simulink model "Rocket"  (R2020a)
settings: Solver=ode4  StartTime=0.0  StopTime=50000  FixedStep=0.5  RelTol=1e-3
undefined symbols (not defined in the file or in its folder): HDBK, MIL
libraries: powerlib_meascontrol x8, simulink x4, aerolibatmos2 x2
settings Model: Creator=j90xb  LastModifiedBy=jasch

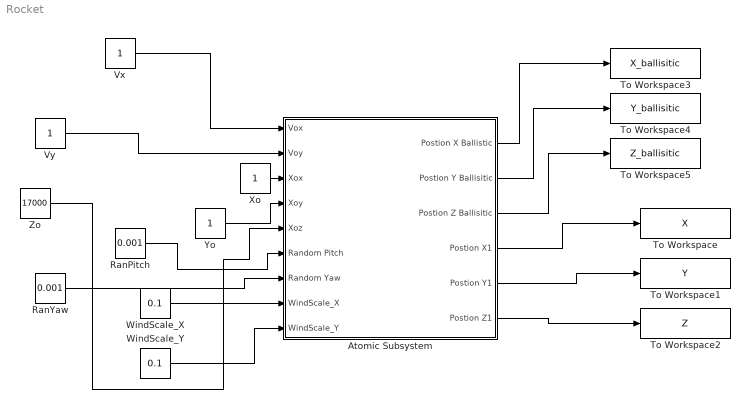
== system Rocket ==
  Atomic Subsystem : Subsystem  TreatAsAtomicUnit=on
  RanPitch : Constant  Value=0.001
  RanYaw : Constant  Value=0.001
  To Workspace : ToWorkspace  VariableName=X  SampleTime=-1
  To Workspace1 : ToWorkspace  VariableName=Y  SampleTime=-1
  To Workspace2 : ToWorkspace  VariableName=Z  SampleTime=-1
  To Workspace3 : ToWorkspace  VariableName=X_ballisitic  SampleTime=-1
  To Workspace4 : ToWorkspace  VariableName=Y_ballisitic  SampleTime=-1
  To Workspace5 : ToWorkspace  VariableName=Z_ballisitic  SampleTime=-1
  Vx : Constant
  Vy : Constant
  WindScale_X : Constant  Value=0.1
  WindScale_Y : Constant  Value=0.1
  Xo : Constant
  Yo : Constant
  Zo : Constant  Value=17000
  wires:
  Vx/1 -> Atomic Subsystem/1(Vox)
  Zo/1 -> Atomic Subsystem/5(Xoz)
  Atomic Subsystem/4(Postion X1) -> To Workspace/1
  Atomic Subsystem/5(Postion Y1) -> To Workspace1/1
  Atomic Subsystem/6(Postion Z1) -> To Workspace2/1
  Atomic Subsystem/1(Postion X Ballistic) -> To Workspace3/1
  Atomic Subsystem/2(Postion Y Ballisitic) -> To Workspace4/1
  Atomic Subsystem/3(Postion Z Ballisitic) -> To Workspace5/1
  Vy/1 -> Atomic Subsystem/2(Voy)
  Xo/1 -> Atomic Subsystem/3(Xox)
  Yo/1 -> Atomic Subsystem/4(Xoy)
  RanPitch/1 -> Atomic Subsystem/6(Random Pitch)
  RanYaw/1 -> Atomic Subsystem/7(Random Yaw)
  WindScale_X/1 -> Atomic Subsystem/8(WindScale_X)
  WindScale_Y/1 -> Atomic Subsystem/9(WindScale_Y)

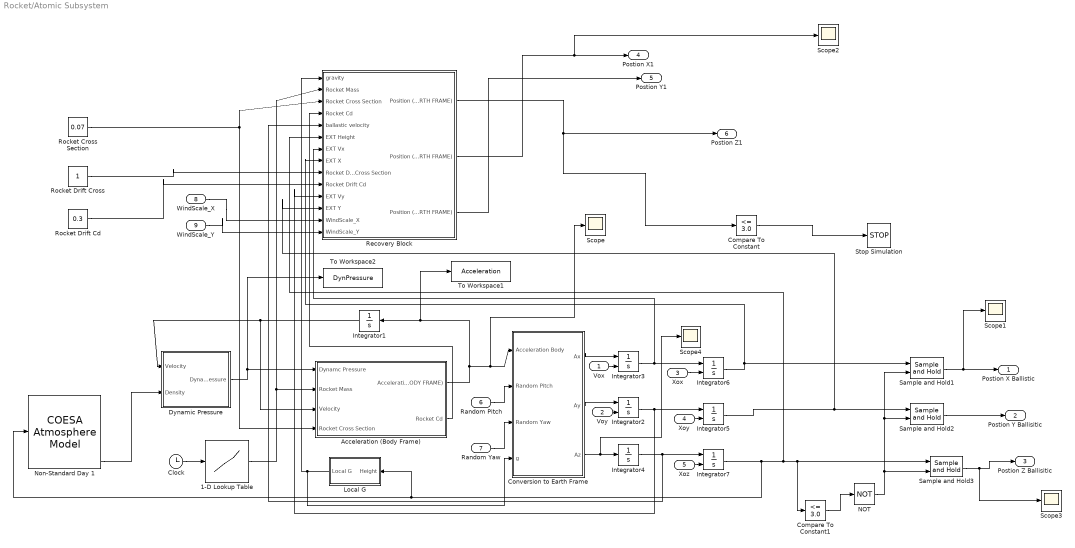
== system Rocket/Atomic Subsystem ==
  Vox : Inport
  Voy : Inport  Port=2
  Xox : Inport  Port=3
  Xoy : Inport  Port=4
  Xoz : Inport  Port=5
  Random Pitch : Inport  Port=6
  Random Yaw : Inport  Port=7
  WindScale_X : Inport  Port=8
  WindScale_Y : Inport  Port=9
  1-D Lookup Table : Lookup_n-D  NumberOfTableDimensions=1  BreakpointsForDimension1=[0,2,5]  Table=[44,30,22]  ExtrapMethod=Clip  UseLastTableValue=on  InternalRulePriority=Speed  RndMeth=Simplest  InputSameDT=on
  Acceleration (Body Frame) : Subsystem  TreatAsAtomicUnit=on
  Clock : Clock
  Compare To Constant : simulink/Logic and Bit Operations/Compare To Constant  relop=<=  const=3.0  OutDataTypeStr=boolean
  Compare To Constant1 : simulink/Logic and Bit Operations/Compare To Constant  relop=<=  const=3.0  OutDataTypeStr=boolean
  Conversion to Earth Frame : Subsystem  TreatAsAtomicUnit=on
  Dynamic Pressure : Subsystem  TreatAsAtomicUnit=on
  Integrator1 : Integrator  InitialCondition=1
  Integrator{2..3,5..7} (5 alike) : Integrator  InitialConditionSource=external
  Integrator4 : Integrator
  Local G : Subsystem
  NOT : Logic  Operator=NOT  IconShape=distinctive  AllPortsSameDT=off  OutDataTypeStr=boolean
  Non-Standard Day 1 : aerolibatmos2/COESA Atmosphere Model  units=Metric (MKS)  spec=MIL-HDBK-310  model=Profile  profile_var=High temperature  profile_percent=1%  profile_alt=5 km (16404 ft)  envelope_var=High temperature  envelope_percent=1%  action=Warning
  Recovery Block : Subsystem  TreatAsAtomicUnit=on
  Rocket Cross Section : Constant  Value=0.07
  Rocket Drift Cd : Constant  Value=0.3
  Rocket Drift Cross : Constant
  Sample and Hold1 : powerlib_meascontrol/Additional Components/Sample and Hold  ic=0  Ts=0
      settings: SourceProductBaseCode=PS
  Sample and Hold2 : powerlib_meascontrol/Additional Components/Sample and Hold  ic=0  Ts=0
      settings: SourceProductBaseCode=PS
  Sample and Hold3 : powerlib_meascontrol/Additional Components/Sample and Hold  ic=0  Ts=0
      settings: SourceProductBaseCode=PS
  Scope{,1..4} (5 alike) : Scope
  Stop Simulation : Stop
  To Workspace1 : ToWorkspace  VariableName=Acceleration  SampleTime=-1
  To Workspace2 : ToWorkspace  VariableName=DynPressure  SampleTime=-1
  Postion X Ballistic : Outport
  Postion Y Ballisitic : Outport  Port=2
  Postion Z Ballisitic : Outport  Port=3
  Postion X1 : Outport  Port=4
  Postion Y1 : Outport  Port=5
  Postion Z1 : Outport  Port=6
  wires:
  Non-Standard Day 1/4 -> Dynamic Pressure/2(Density)
  Dynamic Pressure/1(Dynamic Pressure) -> To Workspace2/1, Acceleration (Body Frame)/1(Dynamc Pressure)
  Acceleration (Body Frame)/1(Acceleration (BODY FRAME)) -> Scope/1, Conversion to Earth Frame/1(Acceleration Body), To Workspace1/1, Integrator1/1
  Conversion to Earth Frame/1(Ax) -> Integrator3/1
  Conversion to Earth Frame/2(Ay) -> Integrator2/1
  Conversion to Earth Frame/3(Az) -> Scope4/1, Integrator4/1
  Integrator3/1 -> Recovery Block/7(EXT Vx), Integrator6/1
  Integrator2/1 -> Recovery Block/11(EXT Vy), Integrator5/1
  Integrator4/1 -> Recovery Block/5(ballastic velocity), Integrator7/1
  Vox/1 -> Integrator3/2
  Voy/1 -> Integrator2/2
  Xox/1 -> Integrator6/2
  Xoy/1 -> Integrator5/2
  Xoz/1 -> Integrator7/2
  Integrator6/1 -> Sample and Hold1/1, Recovery Block/8(EXT X)
  Integrator7/1 -> Local G/1(Height), Non-Standard Day 1/1, Compare To Constant1/1, Sample and Hold3/1, Recovery Block/6(EXT Height)
  Integrator1/1 -> Acceleration (Body Frame)/3(Velocity), Dynamic Pressure/1("Velocity ")
  1-D Lookup Table/1 -> Recovery Block/2(Rocket Mass), Acceleration (Body Frame)/2(Rocket Mass)
  Clock/1 -> 1-D Lookup Table/1
  Local G/1(Local G) -> Conversion to Earth Frame/4(g), Recovery Block/1("gravity ")
  Acceleration (Body Frame)/2(Rocket Cd) -> Recovery Block/4(Rocket Cd)
  Rocket Cross Section/1 -> Acceleration (Body Frame)/4(Rocket Cross Section), Recovery Block/3(Rocket Cross Section)
  Rocket Drift Cd/1 -> Recovery Block/10(Rocket Drift Cd)
  Rocket Drift Cross/1 -> Recovery Block/9(Rocket Drift Cross Section)
  Sample and Hold1/1 -> Scope1/1, Postion X Ballistic/1
  Sample and Hold2/1 -> Postion Y Ballisitic/1
  Sample and Hold3/1 -> Scope3/1, Postion Z Ballisitic/1
  Compare To Constant/1 -> Stop Simulation/1
  NOT/1 -> Sample and Hold1/2, Sample and Hold2/2, Sample and Hold3/2
  Integrator5/1 -> Recovery Block/12(EXT Y), Sample and Hold2/1
  Compare To Constant1/1 -> NOT/1
  Recovery Block/3(Position (Y EARTH FRAME)) -> Postion Y1/1
  Recovery Block/1(Position (Z EARTH FRAME)) -> Compare To Constant/1, Postion Z1/1
  Random Pitch/1 -> Conversion to Earth Frame/2(Random Pitch)
  Random Yaw/1 -> Conversion to Earth Frame/3(Random Yaw)
  WindScale_X/1 -> Recovery Block/13(WindScale_X)
  WindScale_Y/1 -> Recovery Block/14(WindScale_Y)
  Recovery Block/2(Position (X EARTH FRAME)) -> Scope2/1, Postion X1/1

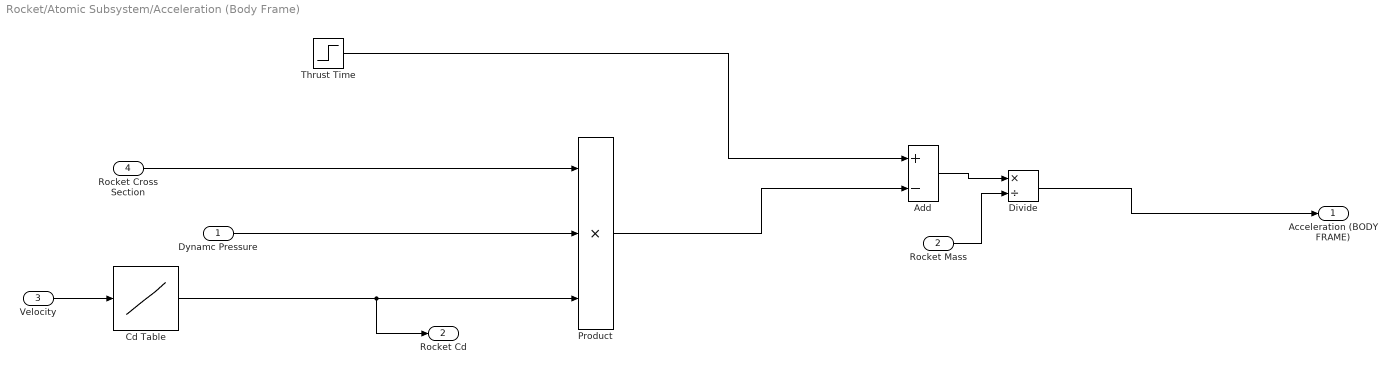
== system Rocket/Atomic Subsystem/Acceleration (Body Frame) ==
  Dynamc Pressure : Inport
  Rocket Mass : Inport  Port=2
  Velocity : Inport  Port=3
  Rocket Cross Section : Inport  Port=4
  Add : Sum  Inputs=+-
  Cd Table : Lookup_n-D  NumberOfTableDimensions=1  BreakpointsForDimension1=[0,0.05,0.1,0.6,0.9,1.1,1.2,2,3,4,5]  Table=[0.48,0.4,0.42,0.4,0.44,0.54,0.52,0.36,0.24,0.18,0.14]  ExtrapMethod=Clip  UseLastTableValue=on  InternalRulePriority=Speed  RndMeth=Simplest  InputSameDT=on
  Divide : Product  Inputs=*/
  Product : Product  Inputs=3
  Thrust Time : Step  Time=6  Before=5000  After=0  SampleTime=0  ZeroCross=off
  Acceleration (BODY FRAME) : Outport
  Rocket Cd : Outport  Port=2
  wires:
  Dynamc Pressure/1 -> Product/2
  Cd Table/1 -> Rocket Cd/1, Product/3
  Rocket Cross Section/1 -> Product/1
  Product/1 -> Add/2
  Add/1 -> Divide/1
  Rocket Mass/1 -> Divide/2
  Thrust Time/1 -> Add/1
  Velocity/1 -> Cd Table/1
  Divide/1 -> Acceleration (BODY FRAME)/1

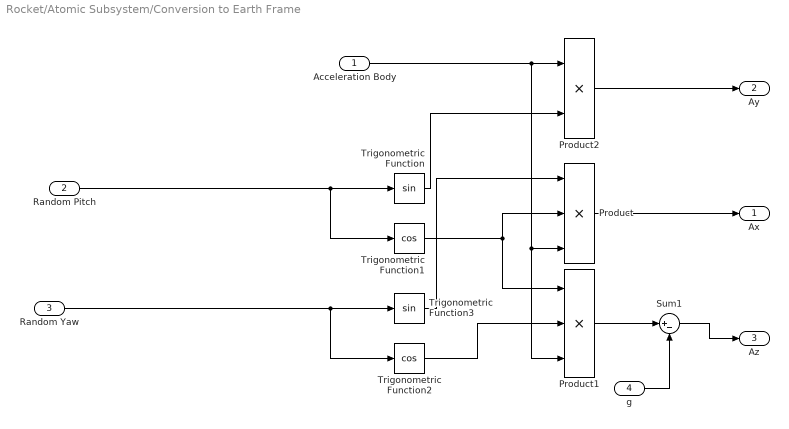
== system Rocket/Atomic Subsystem/Conversion to Earth Frame ==
  Acceleration Body : Inport
  Random Pitch : Inport  Port=2
  Random Yaw : Inport  Port=3
  g : Inport  Port=4
  Product : Product  Inputs=3
  Product1 : Product  Inputs=3
  Product2 : Product
  Sum1 : Sum  Inputs=|+-
  Trigonometric Function : Trigonometry
  Trigonometric Function1 : Trigonometry  Operator=cos
  Trigonometric Function2 : Trigonometry  Operator=cos
  Trigonometric Function3 : Trigonometry
  Ax : Outport
  Ay : Outport  Port=2
  Az : Outport  Port=3
  wires:
  Product/1 -> Ax/1
  Trigonometric Function2/1 -> Product1/2
  Trigonometric Function1/1 -> Product1/1, Product/2
  Trigonometric Function3/1 -> Product/1
  Trigonometric Function/1 -> Product2/2
  Acceleration Body/1 -> Product1/3, Product/3, Product2/1
  Random Pitch/1 -> Trigonometric Function1/1, Trigonometric Function/1
  Random Yaw/1 -> Trigonometric Function2/1, Trigonometric Function3/1
  Product2/1 -> Ay/1
  Product1/1 -> Sum1/1
  Sum1/1 -> Az/1
  g/1 -> Sum1/2

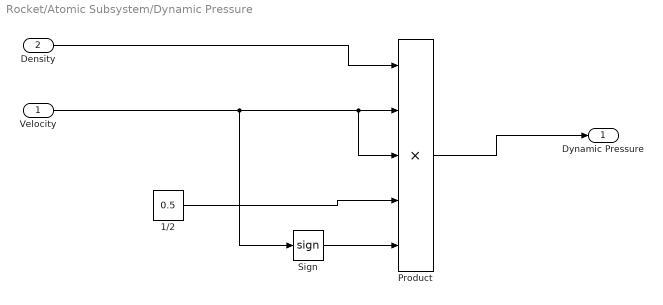
== system Rocket/Atomic Subsystem/Dynamic Pressure ==
  "Velocity " : Inport
  Density : Inport  Port=2
  1/2 : Constant  Value=0.5
  Product : Product  Inputs=5
  Sign : Signum
  Dynamic Pressure : Outport
  wires:
  "Velocity "/1 -> Sign/1, Product/2, Product/3
  Density/1 -> Product/1
  Product/1 -> Dynamic Pressure/1
  1/2/1 -> Product/4
  Sign/1 -> Product/5

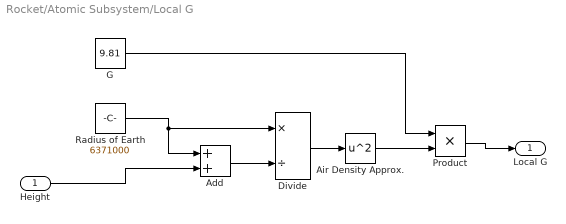
== system Rocket/Atomic Subsystem/Local G ==
  Height : Inport
  Add : Sum
  Air Density Approx. : Math  Operator=square  SignedPower=on  OutMin=0  OutMax=10000  SaturateOnIntegerOverflow=on
  Divide : Product  Inputs=*/
  G : Constant  Value=9.81
  Product : Product
  Radius of Earth : Constant  Value=6371000
  Local G : Outport  VectorParamsAs1DForOutWhenUnconnected=off
  wires:
  Radius of Earth/1 -> Divide/1, Add/1
  Height/1 -> Add/2
  Add/1 -> Divide/2
  Divide/1 -> Air Density Approx./1
  Air Density Approx./1 -> Product/2
  Product/1 -> Local G/1
  G/1 -> Product/1

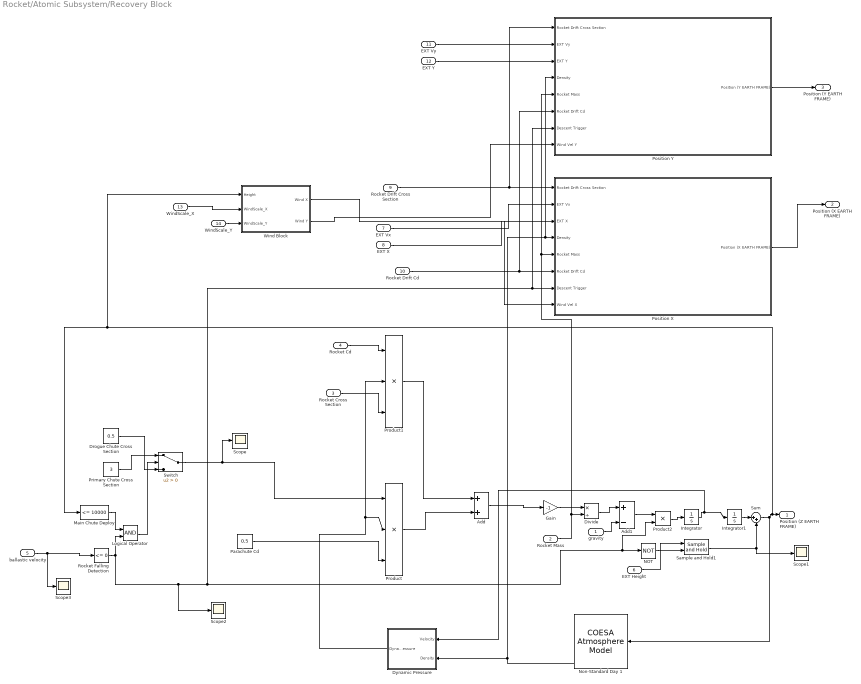
== system Rocket/Atomic Subsystem/Recovery Block ==
  "gravity " : Inport
  Rocket Mass : Inport  Port=2
  Rocket Cross Section : Inport  Port=3
  Rocket Cd : Inport  Port=4
  ballastic velocity : Inport  Port=5
  EXT Height : Inport  Port=6
  EXT Vx : Inport  Port=7
  EXT X : Inport  Port=8
  Rocket Drift Cross Section : Inport  Port=9
  Rocket Drift Cd : Inport  Port=10
  EXT Vy : Inport  Port=11
  EXT Y : Inport  Port=12
  WindScale_X : Inport  Port=13
  WindScale_Y : Inport  Port=14
  Add : Sum
  Add1 : Sum  Inputs=+-
  Divide : Product  Inputs=*/
  Drogue Chute Cross Section : Constant  Value=0.5
  Dynamic Pressure : Subsystem  TreatAsAtomicUnit=on
  Gain : Gain  Gain=-1
  Integrator : Integrator
  Integrator1 : Integrator
  Logical Operator : Logic  AllPortsSameDT=off  OutDataTypeStr=boolean
  Main Chute Deploy : simulink/Logic and Bit Operations/Compare To Constant  relop=<=  const=10000  OutDataTypeStr=boolean
  NOT : Logic  Operator=NOT  IconShape=distinctive  AllPortsSameDT=off  OutDataTypeStr=boolean
  Non-Standard Day 1 : aerolibatmos2/COESA Atmosphere Model  units=Metric (MKS)  spec=MIL-HDBK-310  model=Profile  profile_var=High temperature  profile_percent=1%  profile_alt=5 km (16404 ft)  envelope_var=High temperature  envelope_percent=1%  action=Warning
  Parachute Cd : Constant  Value=0.5
  Position X : Subsystem  TreatAsAtomicUnit=on
  Position Y : Subsystem  TreatAsAtomicUnit=on
  Primary Chute Cross Section : Constant  Value=3
  Product : Product  Inputs=3
  Product1 : Product  Inputs=3
  Product2 : Product
  Rocket Falling Detection : simulink/Logic and Bit Operations/Compare To Constant  relop=<=  const=0  OutDataTypeStr=uint8
  Sample and Hold1 : powerlib_meascontrol/Additional Components/Sample and Hold  ic=10  Ts=0
      settings: SourceProductBaseCode=PS
  Scope{,1..3} (4 alike) : Scope
  Sum : Sum  Inputs=|++
  Switch : Switch  Criteria=u2 > Threshold
  Wind Block : Subsystem  TreatAsAtomicUnit=on
  Position (Z EARTH FRAME) : Outport
  Position (X EARTH FRAME) : Outport  Port=2
  Position (Y EARTH FRAME) : Outport  Port=3
  wires:
  Parachute Cd/1 -> Product/3
  "gravity "/1 -> Add1/2
  Product/1 -> Add/2
  Rocket Cross Section/1 -> Product1/3
  Rocket Cd/1 -> Product1/1
  Dynamic Pressure/1(Dynamic Pressure) -> Product1/2, Product/2
  Non-Standard Day 1/4 -> Position Y/4(Density), Position X/4(Density), Dynamic Pressure/2(Density)
  Product1/1 -> Add/1
  Divide/1 -> Add1/1
  ballastic velocity/1 -> Scope3/1, Rocket Falling Detection/1
  Main Chute Deploy/1 -> Logical Operator/1
  Logical Operator/1 -> Switch/2
  Integrator/1 -> Dynamic Pressure/1("Velocity "), Integrator1/1
  Sample and Hold1/1 -> Scope1/1, Sum/2
  EXT Height/1 -> Sample and Hold1/1
  Rocket Mass/1 -> Divide/2, Position Y/5(Rocket Mass), Position X/5(Rocket Mass)
  Rocket Falling Detection/1 -> Logical Operator/2, Scope2/1, Position Y/7(Descent Trigger), Position X/7(Descent Trigger), NOT/1, Product2/2
  EXT Vx/1 -> Position X/2(EXT Vx)
  EXT X/1 -> Position X/3(EXT X)
  Rocket Drift Cd/1 -> Position Y/6(Rocket Drift Cd), Position X/6(Rocket Drift Cd)
  Add/1 -> Gain/1
  Add1/1 -> Product2/1
  Product2/1 -> Integrator/1
  Integrator1/1 -> Sum/1
  Sum/1 -> Non-Standard Day 1/1, Wind Block/1(Height), Main Chute Deploy/1, Position (Z EARTH FRAME)/1
  NOT/1 -> Sample and Hold1/2
  Gain/1 -> Divide/1
  Position X/1(Position (X EARTH FRAME)) -> Position (X EARTH FRAME)/1
  Position Y/1(Position (Y EARTH FRAME)) -> Position (Y EARTH FRAME)/1
  Rocket Drift Cross Section/1 -> Position Y/1(Rocket Drift Cross Section), Position X/1(Rocket Drift Cross Section)
  EXT Vy/1 -> Position Y/2(EXT Vy)
  EXT Y/1 -> Position Y/3(EXT Y)
  Wind Block/2(Wind Y) -> Position Y/8(Wind Vel Y)
  Wind Block/1(Wind X) -> Position X/8(Wind Vel X)
  Switch/1 -> Scope/1, Product/1
  Drogue Chute Cross Section/1 -> Switch/3
  Primary Chute Cross Section/1 -> Switch/1
  WindScale_X/1 -> Wind Block/2(WindScale_X)
  WindScale_Y/1 -> Wind Block/3(WindScale_Y)

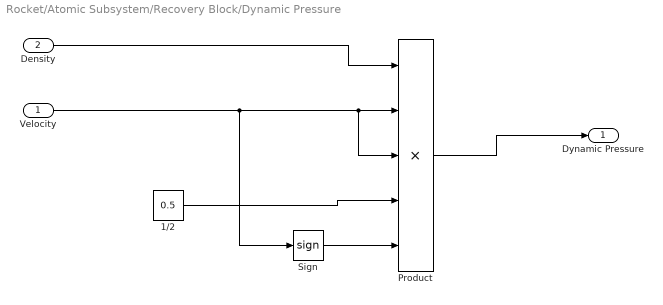
== system Rocket/Atomic Subsystem/Recovery Block/Dynamic Pressure ==
  "Velocity " : Inport
  Density : Inport  Port=2
  1/2 : Constant  Value=0.5
  Product : Product  Inputs=5
  Sign : Signum
  Dynamic Pressure : Outport
  wires:
  "Velocity "/1 -> Sign/1, Product/2, Product/3
  Density/1 -> Product/1
  Product/1 -> Dynamic Pressure/1
  1/2/1 -> Product/4
  Sign/1 -> Product/5

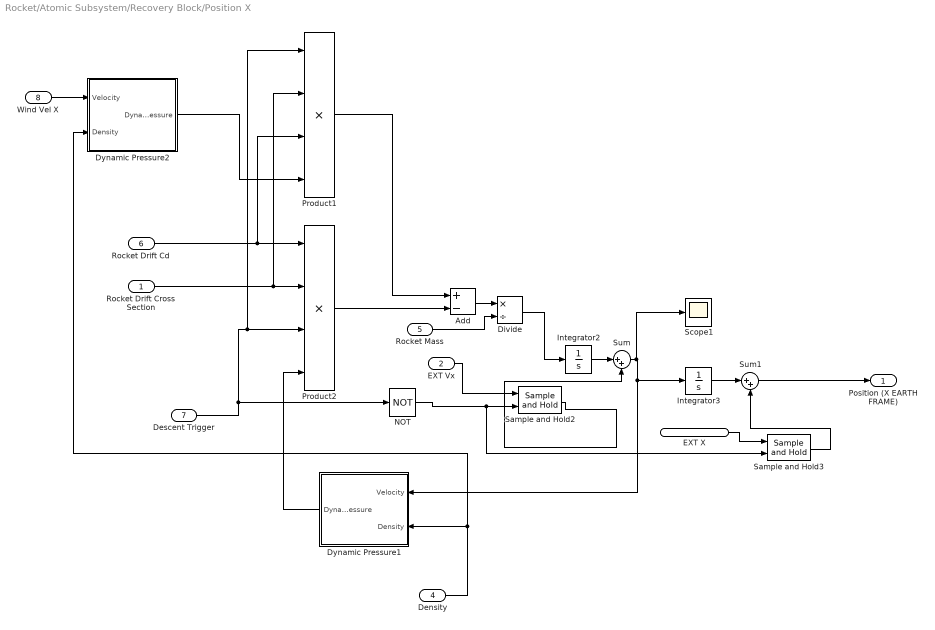
== system Rocket/Atomic Subsystem/Recovery Block/Position X ==
  Rocket Drift Cross Section : Inport
  EXT Vx : Inport  Port=2
  EXT X : Inport  Port=3
  Density : Inport  Port=4
  Rocket Mass : Inport  Port=5
  Rocket Drift Cd : Inport  Port=6
  Descent Trigger : Inport  Port=7
  Wind Vel X : Inport  Port=8
  Add : Sum  Inputs=+-
  Divide : Product  Inputs=*/
  Dynamic Pressure1 : Subsystem  TreatAsAtomicUnit=on
  Dynamic Pressure2 : Subsystem  TreatAsAtomicUnit=on
  Integrator2 : Integrator
  Integrator3 : Integrator
  NOT : Logic  Operator=NOT  IconShape=distinctive  AllPortsSameDT=off  OutDataTypeStr=boolean
  Product1 : Product  Inputs=4
  Product2 : Product  Inputs=4
  Sample and Hold2 : powerlib_meascontrol/Additional Components/Sample and Hold  ic=0  Ts=0
      settings: SourceProductBaseCode=PS
  Sample and Hold3 : powerlib_meascontrol/Additional Components/Sample and Hold  ic=0  Ts=0
      settings: SourceProductBaseCode=PS
  Scope1 : Scope
  Sum : Sum  Inputs=|++
  Sum1 : Sum  Inputs=|++
  Position (X EARTH FRAME) : Outport
  wires:
  Rocket Drift Cd/1 -> Product1/3, Product2/1
  Sample and Hold3/1 -> Sum1/2
  EXT Vx/1 -> Sample and Hold2/1
  Dynamic Pressure1/1(Dynamic Pressure) -> Product2/4
  EXT X/1 -> Sample and Hold3/1
  Density/1 -> Dynamic Pressure2/2(Density), Dynamic Pressure1/2(Density)
  Rocket Mass/1 -> Divide/2
  Descent Trigger/1 -> Product1/1, Product2/3, NOT/1
  Product2/1 -> Add/2
  Dynamic Pressure2/1(Dynamic Pressure) -> Product1/4
  Rocket Drift Cross Section/1 -> Product1/2, Product2/2
  Wind Vel X/1 -> Dynamic Pressure2/1("Velocity ")
  Product1/1 -> Add/1
  Add/1 -> Divide/1
  Divide/1 -> Integrator2/1
  Integrator2/1 -> Sum/1
  Sum/1 -> Scope1/1, Dynamic Pressure1/1("Velocity "), Integrator3/1
  Sample and Hold2/1 -> Sum/2
  NOT/1 -> Sample and Hold2/2, Sample and Hold3/2
  Integrator3/1 -> Sum1/1
  Sum1/1 -> Position (X EARTH FRAME)/1

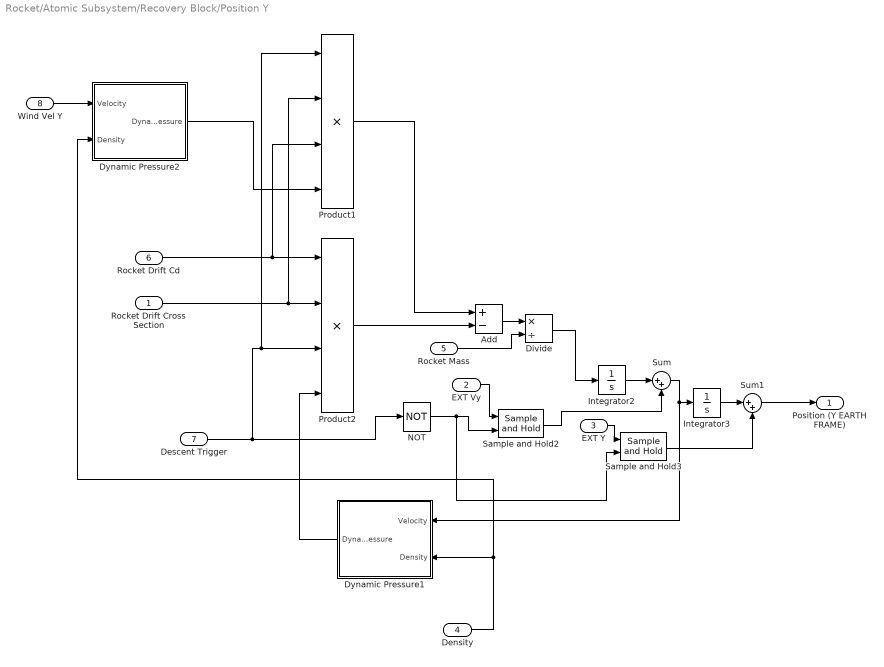
== system Rocket/Atomic Subsystem/Recovery Block/Position Y ==
  Rocket Drift Cross Section : Inport
  EXT Vy : Inport  Port=2
  EXT Y : Inport  Port=3
  Density : Inport  Port=4
  Rocket Mass : Inport  Port=5
  Rocket Drift Cd : Inport  Port=6
  Descent Trigger : Inport  Port=7
  Wind Vel Y : Inport  Port=8
  Add : Sum  Inputs=+-
  Divide : Product  Inputs=*/
  Dynamic Pressure1 : Subsystem  TreatAsAtomicUnit=on
  Dynamic Pressure2 : Subsystem  TreatAsAtomicUnit=on
  Integrator2 : Integrator
  Integrator3 : Integrator
  NOT : Logic  Operator=NOT  IconShape=distinctive  AllPortsSameDT=off  OutDataTypeStr=boolean
  Product1 : Product  Inputs=4
  Product2 : Product  Inputs=4
  Sample and Hold2 : powerlib_meascontrol/Additional Components/Sample and Hold  ic=0  Ts=0
      settings: SourceProductBaseCode=PS
  Sample and Hold3 : powerlib_meascontrol/Additional Components/Sample and Hold  ic=0  Ts=0
      settings: SourceProductBaseCode=PS
  Sum : Sum  Inputs=|++
  Sum1 : Sum  Inputs=|++
  Position (Y EARTH FRAME) : Outport
  wires:
  Sample and Hold2/1 -> Sum/2
  Rocket Drift Cd/1 -> Product1/3, Product2/1
  EXT Vy/1 -> Sample and Hold2/1
  Dynamic Pressure1/1(Dynamic Pressure) -> Product2/4
  EXT Y/1 -> Sample and Hold3/1
  Density/1 -> Dynamic Pressure2/2(Density), Dynamic Pressure1/2(Density)
  Rocket Mass/1 -> Divide/2
  Descent Trigger/1 -> Product1/1, Product2/3, NOT/1
  Product2/1 -> Add/2
  Dynamic Pressure2/1(Dynamic Pressure) -> Product1/4
  Rocket Drift Cross Section/1 -> Product1/2, Product2/2
  Wind Vel Y/1 -> Dynamic Pressure2/1("Velocity ")
  Product1/1 -> Add/1
  Add/1 -> Divide/1
  Divide/1 -> Integrator2/1
  NOT/1 -> Sample and Hold2/2, Sample and Hold3/2
  Integrator2/1 -> Sum/1
  Sum/1 -> Dynamic Pressure1/1("Velocity "), Integrator3/1
  Integrator3/1 -> Sum1/1
  Sum1/1 -> Position (Y EARTH FRAME)/1
  Sample and Hold3/1 -> Sum1/2

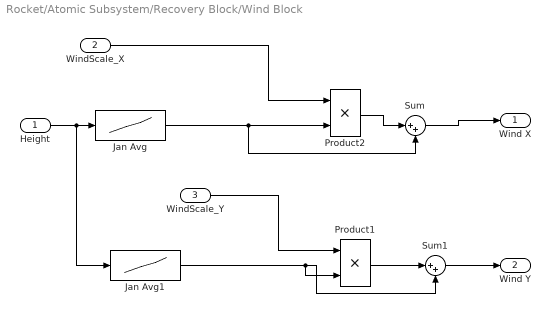
== system Rocket/Atomic Subsystem/Recovery Block/Wind Block ==
  Height : Inport
  WindScale_X : Inport  Port=2
  WindScale_Y : Inport  Port=3
  Jan Avg : Lookup_n-D  NumberOfTableDimensions=1  BreakpointsForDimension1=[0,5000,10000,15000,20000,24000,100000]  Table=[2,17,30,22,5,2,0]  InterpMethod=Cubic spline  ExtrapMethod=Clip  UseLastTableValue=on  InternalRulePriority=Speed  RndMeth=Simplest  InputSameDT=on
  Jan Avg1 : Lookup_n-D  NumberOfTableDimensions=1  BreakpointsForDimension1=[0,5000,10000,15000,20000,24000,100000]  Table=[2,17,30,22,5,2,0]  InterpMethod=Cubic spline  ExtrapMethod=Clip  UseLastTableValue=on  InternalRulePriority=Speed  RndMeth=Simplest  InputSameDT=on
  Product1 : Product
  Product2 : Product
  Sum : Sum  Inputs=|++
  Sum1 : Sum  Inputs=|++
  Wind X : Outport
  Wind Y : Outport  Port=2
  wires:
  Height/1 -> Jan Avg1/1, Jan Avg/1
  WindScale_X/1 -> Product2/1
  Jan Avg/1 -> Sum/2, Product2/2
  WindScale_Y/1 -> Product1/1
  Jan Avg1/1 -> Sum1/2, Product1/2
  Product2/1 -> Sum/1
  Sum/1 -> Wind X/1
  Product1/1 -> Sum1/1
  Sum1/1 -> Wind Y/1

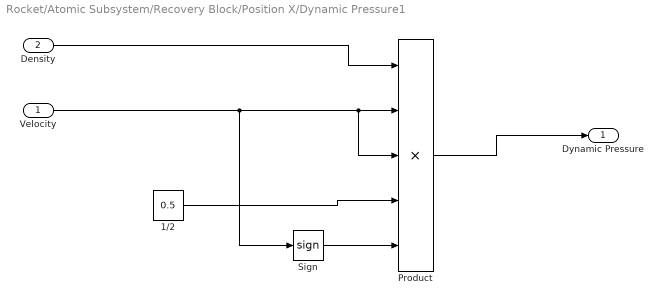
== system Rocket/Atomic Subsystem/Recovery Block/Position X/Dynamic Pressure1 ==
  "Velocity " : Inport
  Density : Inport  Port=2
  1/2 : Constant  Value=0.5
  Product : Product  Inputs=5
  Sign : Signum
  Dynamic Pressure : Outport
  wires:
  "Velocity "/1 -> Sign/1, Product/2, Product/3
  Density/1 -> Product/1
  Product/1 -> Dynamic Pressure/1
  1/2/1 -> Product/4
  Sign/1 -> Product/5

== system Rocket/Atomic Subsystem/Recovery Block/Position X/Dynamic Pressure2 ==
  "Velocity " : Inport
  Density : Inport  Port=2
  1/2 : Constant  Value=0.5
  Product : Product  Inputs=5
  Sign : Signum
  Dynamic Pressure : Outport
  wires:
  "Velocity "/1 -> Sign/1, Product/2, Product/3
  Density/1 -> Product/1
  Product/1 -> Dynamic Pressure/1
  1/2/1 -> Product/4
  Sign/1 -> Product/5

== system Rocket/Atomic Subsystem/Recovery Block/Position Y/Dynamic Pressure1 ==
  "Velocity " : Inport
  Density : Inport  Port=2
  1/2 : Constant  Value=0.5
  Product : Product  Inputs=5
  Sign : Signum
  Dynamic Pressure : Outport
  wires:
  "Velocity "/1 -> Sign/1, Product/2, Product/3
  Density/1 -> Product/1
  Product/1 -> Dynamic Pressure/1
  1/2/1 -> Product/4
  Sign/1 -> Product/5

== system Rocket/Atomic Subsystem/Recovery Block/Position Y/Dynamic Pressure2 ==
  "Velocity " : Inport
  Density : Inport  Port=2
  1/2 : Constant  Value=0.5
  Product : Product  Inputs=5
  Sign : Signum
  Dynamic Pressure : Outport
  wires:
  "Velocity "/1 -> Sign/1, Product/2, Product/3
  Density/1 -> Product/1
  Product/1 -> Dynamic Pressure/1
  1/2/1 -> Product/4
  Sign/1 -> Product/5
